simulink model "Modelo"  (R2015a)
settings: Solver=ode45  StartTime=0.0  StopTime=Tsim  RelTol=1e-4
undefined symbols (not defined in the file or in its folder): C, G, vdes
settings Model: Creator=pedro  LastModifiedBy=gabas_000
settings OptimizationCC: ExpressionDepthLimit=2147483647
settings DebuggingCC: UnderspecifiedInitializationDetection=Classic  MergeDetectMultiDrivingBlocksExec=none  SolverPrmCheckMsg=warning  StateNameClashWarn=warning

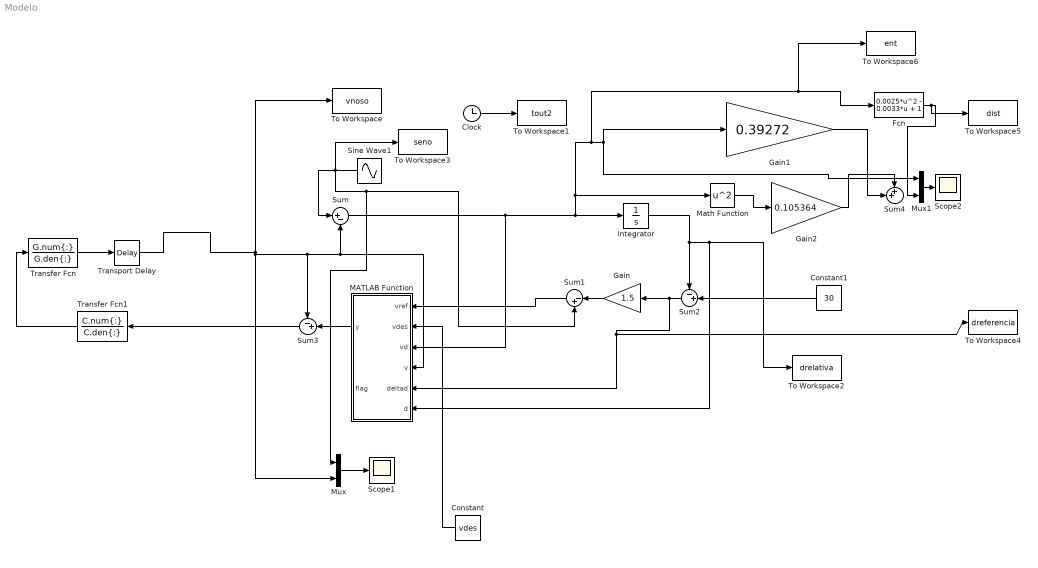
== system Modelo ==
  Clock : Clock
  Constant : Constant  Value=vdes
  Constant1 : Constant  Value=30
  Fcn : Fcn  Expr=0.0025*u^2 - 0.0033*u + 1
  Gain : Gain  Gain=1.5
  Gain1 : Gain  Gain=0.39272
  Gain2 : Gain  Gain=0.105364
  Integrator : Integrator
  MATLAB Function : MATLAB Function  TreatAsAtomicUnit=on
  Math Function : Math  Operator=square  SaturateOnIntegerOverflow=on
  Mux : Mux  Inputs=2
  Mux1 : Mux  Inputs=2
  Scope1 : Scope
  Scope2 : Scope
  Sine Wave1 : Sin  Amplitude=1.39  Bias=13.9  Frequency=.001  Phase=27
  Sum : Sum  Inputs=|+-
  Sum1 : Sum  Inputs=|-+
  Sum2 : Sum  Inputs=-+|
  Sum3 : Sum  Inputs=-+|
  Sum4 : Sum  Inputs=++|
  To Workspace : ToWorkspace  VariableName=vnoso  SampleTime=-1
  To Workspace1 : ToWorkspace  VariableName=tout2  SampleTime=-1
  To Workspace2 : ToWorkspace  VariableName=drelativa  SampleTime=-1
  To Workspace3 : ToWorkspace  VariableName=seno  SampleTime=-1
  To Workspace4 : ToWorkspace  VariableName=dreferencia  SampleTime=-1
  To Workspace5 : ToWorkspace  VariableName=dist  SampleTime=-1
  To Workspace6 : ToWorkspace  VariableName=ent  SampleTime=-1
  Transfer Fcn : TransferFcn  Numerator=G.num{:}  Denominator=G.den{:}
  Transfer Fcn1 : TransferFcn  Numerator=C.num{:}  Denominator=C.den{:}
  Transport Delay : TransportDelay  DelayTime=G.InputDelay
  wires:
  Integrator/1 -> MATLAB Function/6(d), To Workspace2/1, Sum2/1
  Sum2/1 -> To Workspace4/1, MATLAB Function/5(deltad), Gain/1
  Gain/1 -> Sum1/1
  MATLAB Function/1(y) -> Sum3/2
  Sum1/1 -> MATLAB Function/1(vref)
  Sum/1 -> MATLAB Function/3(vd), To Workspace6/1, Fcn/1, Mux1/1, Gain1/1, Math Function/1, Integrator/1
  Math Function/1 -> Gain2/1
  Constant/1 -> MATLAB Function/2(vdes)
  Sine Wave1/1 -> To Workspace3/1, Mux/1, Sum1/2, Sum/1
  Clock/1 -> To Workspace1/1
  Mux/1 -> Scope1/1
  Transfer Fcn/1 -> Transport Delay/1
  Sum3/1 -> Transfer Fcn1/1
  Transfer Fcn1/1 -> Transfer Fcn/1
  Fcn/1 -> To Workspace5/1, Mux1/2
  Gain2/1 -> Sum4/1
  Gain1/1 -> Sum4/2
  Mux1/1 -> Scope2/1
  Constant1/1 -> Sum2/2
  Transport Delay/1 -> Sum3/1, MATLAB Function/4(v), Sum/2, Mux/2, To Workspace/1

== matlab function Modelo/MATLAB Function ==
  data: vref input; vdes input; y output; vd input; v input; deltad input; d input; flag output
function [y,flag]  = fcn(vref, vdes, vd, v, deltad,d)
%#codegen
%if(deltad<0)
%    y=vdes;
%end

%if(deltad>0 && v<vref)
%    y=vref;
%end


% if(deltad<0)
%     y=vdes;
% elseif(v<vref)
%     y=min(vdes, vref);
% elseif(vd<0)
%     y=min(vdes, vref);
% else
%     y=vdes;
% end

if(d >=10)
    flag = 1;
    if(deltad<0)
        y=vdes;
    else
        if(v<vref)
            y=min(vdes, vref);
        else
            if(vd < 0)
                y=min(vdes, vref);
            else
                y = vdes;
            end
        end
    end
else
    y = 0;
    flag = 0;
end
